simulink model "UnifiedPowerFlowController"  (R2024a)
settings: Solver=FixedStepDiscrete  StartTime=0.0  StopTime=0.8  FixedStep=Ts  RelTol=1e-3
PreLoadFcn:
  | Ts=1/512/60;
undefined symbols (not defined in the file or in its folder): DiscIntNeverNeededParam
libraries: spsabctodq0Lib x10, spsMeanVariableFrequencyLib x10, spsThreeLevelBridgeLib x8, spsVoltageMeasurementLib x8, spsZigzagPhaseShiftingTransformerLib x8, spsCurrentMeasurementLib x6, spsSecondOrderFilterLib x5, spsThreePhaseVIMeasurementLib x4, spsSeriesRLCBranchLib x4, spsDistributedParametersLineLib x3, spsPowerPositiveSequenceLib x3, spsThreePhaseSourceLib x2
(part 3 of 7)

== system UnifiedPowerFlowController/UPFC Controller/SE Control (SSSC)/PLL1 ==
  Vabc (pu) : Inport  PortDimensions=3
  Constant4 : Constant  Value=2*pi
  Correction for delay : Gain  Gain=Nstep*Ts*2*pi  SaturateOnIntegerOverflow=on  OutDataTypeStr=Inherit: Same as input  ParamDataTypeStr=Inherit: Same as input
  Discrete PI Controller : Subsystem  DialogController=POWERSYS.PowerSysDialog  mask(Discrete PI Controller){Kp=Kp, Ki=Ki, Par_Limits=2*pi*Finit*[1.25 0.75], Init=2*pi*Finit, Ts=Ts}
      mask prompts: Kp "Proportional gain (Kp):"; Ki "Integral gain (Ki):"; Par_Limits "Output limits: [ Upper   Lower ]"; Init "Output initial value:"; Ts "Sample time:"
      mask help: This block implements a discrete PI controller.
      mask init:
      | UpperLimit=Par_Limits(1);
      | LowerLimit=Par_Limits(2);
      | power_initmask();
      mask Help: This block is part of a subset of blocks in the Extras library that does not have documentation associated with it, other than the block mask description.
      mask Display: disp('PI');
  Discrete Rate Limiter : Subsystem  DialogController=POWERSYS.PowerSysDialog  mask(Discrete Rate Limiter){R=10, F=-10, Vinit=Finit, Ts=Ts}
      mask prompts: R "Rising slew rate:"; F "Falling slew rate:"; Vinit "Initial input:"; Ts "Sample time:"
      mask help: DISCRETE BLOCK : Limit rising and falling rates of signal
      mask init:
      | UpperLimit=R*Ts;
      | LowerLimit=F*Ts;
      | power_initmask();
      mask Help: This block is part of a subset of blocks in the Extras library that does not have documentation associated with it, other than the block mask description.
      mask Display: disp('Discrete\nRate\nLimiter')
  Discrete-Time Integrator : DiscreteIntegrator  InitialCondition=Phase_Init*pi/180  SampleTime=Ts  ICPrevOutput=DiscIntNeverNeededParam  ICPrevScaledInput=DiscIntNeverNeededParam
  Gain10 : Gain  Gain=1/2/pi  SaturateOnIntegerOverflow=on  OutDataTypeStr=Inherit: Same as input  ParamDataTypeStr=Inherit: Same as input
  Math Function : Math  Operator=mod  SignedPower=on
  Mean (Variable Frequency) : spsMeanVariableFrequencyLib/Mean (Variable Frequency)  Finit=Finit  Fmin=45  Vinit=0  Ts=Ts
  Second-Order Filter : spsSecondOrderFilterLib/Second-Order Filter  FilterType=Lowpass  Fo=25  Zeta=0.707  Ts=Ts  Initialize=on  Vac_Init=[0 -25 60]  Vdc_Init=Finit  PlotResponse=off  FreqRange=[0, 500, 1]
  Selector : Selector  InputPortWidth=3  IndexOptions=Index vector (dialog)  Indices=2  OutputSizes=1
  Sum : Sum  InputSameDT=on  SaturateOnIntegerOverflow=on  OutDataTypeStr=Inherit: Same as first input
  Unit Delay : UnitDelay  InitialCondition=Finit  SampleTime=Ts  HasFrameUpgradeWarning=on
  abc to dq0 : spsabctodq0Lib/abc to dq0  Alignment=90 degrees behind phase A axis
  Freq : Outport  VectorParamsAs1DForOutWhenUnconnected=off
  wt : Outport  Port=2  VectorParamsAs1DForOutWhenUnconnected=off
  wires:
  Sum/1 -> wt/1
  Selector/1 -> Mean (Variable Frequency)/2  "Vq"
  Second-Order Filter/1 -> Unit Delay/1
  Unit Delay/1 -> Correction for delay/1, Mean (Variable Frequency)/1, Freq/1
  Discrete Rate Limiter/1(Out) -> Second-Order Filter/1
  Gain10/1 -> Discrete Rate Limiter/1(In)
  Discrete PI Controller/1(Out) -> Gain10/1, Discrete-Time Integrator/1  "W"
  Math Function/1 -> abc to dq0/2, Sum/2
  Discrete-Time Integrator/1 -> Math Function/1
  Constant4/1 -> Math Function/2
  abc to dq0/1 -> Selector/1
  Vabc (pu)/1 -> abc to dq0/1
  Mean (Variable Frequency)/1 -> Discrete PI Controller/1(Error)
  Correction for delay/1 -> Sum/1

== system UnifiedPowerFlowController/UPFC Controller/SE Control (SSSC)/determine +pi//2 or -pi//2 phase shift ==
  Vref : Inport
  Delta_Alpha : Inport  Port=2
  Constant1 : Constant  Value=pi/2
  Product : Product  SaturateOnIntegerOverflow=on  OutDataTypeStr=Inherit: Same as first input
  Sum1 : Sum  SaturateOnIntegerOverflow=on
  Switch : Switch  InputSameDT=off
  Vdcmin1 : Constant
  Vdcmin2 : Constant  Value=-1
  Alpha : Outport  VectorParamsAs1DForOutWhenUnconnected=off
  wires:
  Product/1 -> Alpha/1
  Sum1/1 -> Product/2
  Switch/1 -> Product/1
  Vdcmin2/1 -> Switch/3
  Delta_Alpha/1 -> Sum1/2
  Vref/1 -> Switch/2
  Vdcmin1/1 -> Switch/1
  Constant1/1 -> Sum1/1

== system UnifiedPowerFlowController/UPFC Controller/SE Control (UPFC)/Current Regulators ==
  note: Current Regulators
  note: =================
  Id_Iq_Ref : Inport  PortDimensions=2
  Id_Iq : Inport  Port=2  PortDimensions=2
  Demux : Demux  Outputs=2
      settings: DisplayOption=none
  Demux1 : Demux  Outputs=2
      settings: DisplayOption=none
  Id PID : Subsystem  DialogController=POWERSYS.PowerSysDialog  mask(Discrete PID Controller){Kp=Kp, Ki=Ki, Kd=Kd, TcD=TcD, Par_Limits=Par_Limits, Init=Init, Ts=Ts}
      mask prompts: Kp "Proportional gain (Kp):"; Ki "Integral gain (Ki):"; Kd "Derivative gain (Kd):"; TcD "Time constant for derivative (s):"; Par_Limits "Output limits: [ Upper   Lower ]"; Init "Output initial value:"; Ts "Sample time:"
      mask help: This block implements a discrete PID controller.
      mask init:
      | UpperLimit=Par_Limits(1);
      | LowerLimit=Par_Limits(2);
      | power_initmask();
      mask Help: This block is part of a subset of blocks in the Extras library that does not have documentation associated with it, other than the block mask description.
      mask Display: disp('PID');
  Id PID1 : Subsystem  DialogController=POWERSYS.PowerSysDialog  mask(Discrete PID Controller){Kp=Kp, Ki=Ki, Kd=Kd, TcD=TcD, Par_Limits=Par_Limits, Init=Init, Ts=Ts}
      mask prompts: Kp "Proportional gain (Kp):"; Ki "Integral gain (Ki):"; Kd "Derivative gain (Kd):"; TcD "Time constant for derivative (s):"; Par_Limits "Output limits: [ Upper   Lower ]"; Init "Output initial value:"; Ts "Sample time:"
      mask help: This block implements a discrete PID controller.
      mask init:
      | UpperLimit=Par_Limits(1);
      | LowerLimit=Par_Limits(2);
      | power_initmask();
      mask Help: This block is part of a subset of blocks in the Extras library that does not have documentation associated with it, other than the block mask description.
      mask Display: disp('PID');
  Mux : Mux  Inputs=2
  Sum : Sum  Inputs=|-+  InputSameDT=on  SaturateOnIntegerOverflow=on  OutDataTypeStr=Inherit: Same as first input
  Sum1 : Sum  Inputs=|-+  InputSameDT=on  SaturateOnIntegerOverflow=on  OutDataTypeStr=Inherit: Same as first input
  VdVq* : Outport  VectorParamsAs1DForOutWhenUnconnected=off
  wires:
  Id_Iq/1 -> Demux/1
  Demux/1 -> Sum/1  "Id"
  Demux1/1 -> Sum/2  "Id_Ref"
  Demux/2 -> Sum1/1  "Iq"
  Sum1/1 -> Id PID1/1(Error)
  Demux1/2 -> Sum1/2  "Iq_Ref"
  Id_Iq_Ref/1 -> Demux1/1
  Mux/1 -> VdVq*/1
  Id PID/1(Out) -> Mux/1  "Vd"
  Id PID1/1(Out) -> Mux/2  "Vq"
  Sum/1 -> Id PID/1(Error)

== system UnifiedPowerFlowController/UPFC Controller/SE Control (UPFC)/Firing Pulses Generator ==
  Sigma : Inport  PortDimensions=1
  D_Alpha : Inport  Port=2  PortDimensions=1
  Alpha : Inport  Port=3  PortDimensions=1
  wt : Inport  Port=4  PortDimensions=1
  " Deg->Rad" : Gain  Gain=pi/180  SaturateOnIntegerOverflow=on  OutDataTypeStr=Inherit: Same as input  ParamDataTypeStr=Inherit: Same as input
  Bridge 1D : Subsystem
  "Bridge 1Y " : Subsystem
  Bridge 2D : Subsystem
  Bridge 2Y : Subsystem
  Constant : Constant  Value=[0 -30 -15 -45]*pi/180 + 7.5*pi/180
  Deg->Rad : Gain  Gain=pi/180  SaturateOnIntegerOverflow=on  OutDataTypeStr=Inherit: Same as input  ParamDataTypeStr=Inherit: Same as input
  "Deg->Rad " : Gain  Gain=pi/180  SaturateOnIntegerOverflow=on  OutDataTypeStr=Inherit: Same as input  ParamDataTypeStr=Inherit: Same as input
  Demux : Demux
      settings: DisplayOption=none
  Mux : Mux  Inputs=[12 12 12 12]
  Sum : Sum  InputSameDT=on  SaturateOnIntegerOverflow=on  OutDataTypeStr=Inherit: Same as first input
  Pulses : Outport  VectorParamsAs1DForOutWhenUnconnected=off
  wires:
  Alpha/1 -> Deg->Rad/1
  Constant/1 -> Sum/2
  Sum/1 -> Demux/1
  "Bridge 1Y "/1(Pulses) -> Mux/1
  Mux/1 -> Pulses/1
  Demux/1 -> "Bridge 1Y "/1(wt)
  Sigma/1 -> "Deg->Rad "/1
  Demux/2 -> Bridge 1D/1(wt)
  Demux/3 -> Bridge 2Y/1(wt)
  Demux/4 -> Bridge 2D/1(wt)
  Deg->Rad/1 -> "Bridge 1Y "/2(Alpha), Bridge 1D/2(Alpha), Bridge 2Y/2(Alpha), Bridge 2D/2(Alpha)
  "Deg->Rad "/1 -> "Bridge 1Y "/3(Sigma), Bridge 1D/3(Sigma), Bridge 2Y/3(Sigma), Bridge 2D/3(Sigma)
  " Deg->Rad"/1 -> Bridge 2D/4(D_Alpha), Bridge 2Y/4(D_Alpha), Bridge 1D/4(D_Alpha), "Bridge 1Y "/4(D_Alpha)
  D_Alpha/1 -> " Deg->Rad"/1
  Bridge 1D/1(Pulses) -> Mux/2
  Bridge 2Y/1(Pulses) -> Mux/3
  Bridge 2D/1(Pulses) -> Mux/4
  wt/1 -> Sum/1

== system UnifiedPowerFlowController/UPFC Controller/SE Control (UPFC)/Mag//rho and sigma computation ==
  VdVq : Inport
  VdcPM_SE : Inport  Port=2  PortDimensions=2
  Demux : Demux  Outputs=2
      settings: DisplayOption=none
  Sigma Computation : Subsystem
  Sum1 : Sum  Inputs=1  InputSameDT=on  SaturateOnIntegerOverflow=on  OutDataTypeStr=Inherit: Same as first input
  Vd_Vq--> Mag,rho : Subsystem
  Sigma : Outport  VectorParamsAs1DForOutWhenUnconnected=off
  rho : Outport  Port=2  VectorParamsAs1DForOutWhenUnconnected=off
  tag scope: Mag_rho_SE=global, Sigma_SE=global
  wires:
  Demux/1 -> Sigma Computation/1(Mag (pu))
  VdcPM_SE/1 -> Sum1/1
  Vd_Vq--> Mag,rho/1(Mag_rho) -> Demux/1, [Mag_rho_SE]
  Sum1/1 -> Sigma Computation/2(Vdc (V))
  VdVq/1 -> Vd_Vq--> Mag,rho/1(Vd_Vq)
  Demux/2 -> rho/1
  Sigma Computation/1(sigma (deg)) -> Sigma/1, [Sigma_SE]

== system UnifiedPowerFlowController/UPFC Controller/SE Control (UPFC)/Measurement System ==
  Freq : Inport  PortDimensions=1
  wt : Inport  Port=2  PortDimensions=1
  Vabc : Inport  Port=3  PortDimensions=3
  Iabc : Inport  Port=4  PortDimensions=3
  PQ Computaion : Subsystem
  Selector : Selector  InputPortWidth=3  IndexOptions=Index vector (dialog)  Indices=[1 2]  OutputSizes=1
  Voltage Measurement : Subsystem  mask(Discrete 3-phase PLL-Driven Positive-Sequence Fundamental Value){Finit=60, Par_Init=[1.0001 -1.5], Ts=Ts}
      mask prompts: Finit "Initial fundamental frequency (Hz):"; Par_Init "Initial input (positive component): [ Mag  Phase-relative-to-PLL(degrees) ]"; Ts "Sample time:"
      mask help:
      | For a supplied fundamental frequency (port Freq), this discrete block computes  the positive-sequence component (Magnitude and Phase)  of a set of three balanced or unbalanced signals (port abc) which may contain harmonics.
      |  Input port "Sin_Cos" (a two-dimension signal) provides the reference frame required for the computation..
      |  First and second outputs return respectively the magnitude and phase (in degrees relative to the PLL phase)) of the fundamental.
      | For the first cycle of simulation, the outputs are held constant to the values specified by the parameter "Initial input".
      mask init:
      | Real_Init=Par_Init(1)*cos(pi/180*Par_Init(2));
      | Imag_Init=Par_Init(1)*sin(pi/180*Par_Init(2));
  Voltage Measurement1 : Subsystem  mask(Discrete 3-phase PLL-Driven Positive-Sequence Fundamental Value){Finit=60, Par_Init=[8.7 0], Ts=Ts}
      mask prompts: Finit "Initial fundamental frequency (Hz):"; Par_Init "Initial input (positive component): [ Mag  Phase-relative-to-PLL(degrees) ]"; Ts "Sample time:"
      mask help:
      | For a supplied fundamental frequency (port Freq), this discrete block computes  the positive-sequence component (Magnitude and Phase)  of a set of three balanced or unbalanced signals (port abc) which may contain harmonics.
      |  Input port "Sin_Cos" (a two-dimension signal) provides the reference frame required for the computation..
      |  First and second outputs return respectively the magnitude and phase (in degrees relative to the PLL phase)) of the fundamental.
      | For the first cycle of simulation, the outputs are held constant to the values specified by the parameter "Initial input".
      mask init:
      | Real_Init=Par_Init(1)*cos(pi/180*Par_Init(2));
      | Imag_Init=Par_Init(1)*sin(pi/180*Par_Init(2));
  abc to dq0 : spsabctodq0Lib/abc to dq0  Alignment=90 degrees behind phase A axis
  PQ : Outport  VectorParamsAs1DForOutWhenUnconnected=off
  Vd_Vq : Outport  Port=2  VectorParamsAs1DForOutWhenUnconnected=off
  Id_Iq : Outport  Port=3  VectorParamsAs1DForOutWhenUnconnected=off
  wires:
  Voltage Measurement/1(VdVq) -> Vd_Vq/1, PQ Computaion/1(Vd_Vq)
  Freq/1 -> Voltage Measurement/1(Freq), Voltage Measurement1/1(Freq)
  Iabc/1 -> Voltage Measurement1/3(abc), abc to dq0/1
  Vabc/1 -> Voltage Measurement/3(abc)
  PQ Computaion/1(P_Q) -> PQ/1
  abc to dq0/1 -> Selector/1
  Selector/1 -> Id_Iq/1
  Voltage Measurement1/1(IdIq) -> PQ Computaion/2(Id_Iq)
  wt/1 -> abc to dq0/2, Voltage Measurement1/2(wt), Voltage Measurement/2(wt)

== system UnifiedPowerFlowController/UPFC Controller/SE Control (UPFC)/PLL1 ==
  Vabc (pu) : Inport  PortDimensions=3
  Constant4 : Constant  Value=2*pi
  Correction for delay : Gain  Gain=Nstep*Ts*2*pi  SaturateOnIntegerOverflow=on  OutDataTypeStr=Inherit: Same as input  ParamDataTypeStr=Inherit: Same as input
  Discrete PI Controller : Subsystem  DialogController=POWERSYS.PowerSysDialog  mask(Discrete PI Controller){Kp=Kp, Ki=Ki, Par_Limits=2*pi*Finit*[1.25 0.75], Init=2*pi*Finit, Ts=Ts}
      mask prompts: Kp "Proportional gain (Kp):"; Ki "Integral gain (Ki):"; Par_Limits "Output limits: [ Upper   Lower ]"; Init "Output initial value:"; Ts "Sample time:"
      mask help: This block implements a discrete PI controller.
      mask init:
      | UpperLimit=Par_Limits(1);
      | LowerLimit=Par_Limits(2);
      | power_initmask();
      mask Help: This block is part of a subset of blocks in the Extras library that does not have documentation associated with it, other than the block mask description.
      mask Display: disp('PI');
  Discrete Rate Limiter : Subsystem  DialogController=POWERSYS.PowerSysDialog  mask(Discrete Rate Limiter){R=10, F=-10, Vinit=Finit, Ts=Ts}
      mask prompts: R "Rising slew rate:"; F "Falling slew rate:"; Vinit "Initial input:"; Ts "Sample time:"
      mask help: DISCRETE BLOCK : Limit rising and falling rates of signal
      mask init:
      | UpperLimit=R*Ts;
      | LowerLimit=F*Ts;
      | power_initmask();
      mask Help: This block is part of a subset of blocks in the Extras library that does not have documentation associated with it, other than the block mask description.
      mask Display: disp('Discrete\nRate\nLimiter')
  Discrete-Time Integrator : DiscreteIntegrator  InitialCondition=Phase_Init*pi/180  SampleTime=Ts  ICPrevOutput=DiscIntNeverNeededParam  ICPrevScaledInput=DiscIntNeverNeededParam
  Gain10 : Gain  Gain=1/2/pi  SaturateOnIntegerOverflow=on  OutDataTypeStr=Inherit: Same as input  ParamDataTypeStr=Inherit: Same as input
  Math Function : Math  Operator=mod  SignedPower=on
  Mean (Variable Frequency) : spsMeanVariableFrequencyLib/Mean (Variable Frequency)  Finit=Finit  Fmin=45  Vinit=0  Ts=Ts
  Second-Order Filter : spsSecondOrderFilterLib/Second-Order Filter  FilterType=Lowpass  Fo=25  Zeta=0.707  Ts=Ts  Initialize=on  Vac_Init=[0 -25 60]  Vdc_Init=Finit  PlotResponse=off  FreqRange=[0, 500, 1]
  Selector : Selector  InputPortWidth=3  IndexOptions=Index vector (dialog)  Indices=2  OutputSizes=1
  Sum : Sum  InputSameDT=on  SaturateOnIntegerOverflow=on  OutDataTypeStr=Inherit: Same as first input
  Unit Delay : UnitDelay  InitialCondition=Finit  SampleTime=Ts  HasFrameUpgradeWarning=on
  abc to dq0 : spsabctodq0Lib/abc to dq0  Alignment=90 degrees behind phase A axis
  Freq : Outport  VectorParamsAs1DForOutWhenUnconnected=off
  wt : Outport  Port=2  VectorParamsAs1DForOutWhenUnconnected=off
  wires:
  Sum/1 -> wt/1
  Selector/1 -> Mean (Variable Frequency)/2  "Vq"
  Second-Order Filter/1 -> Unit Delay/1
  Unit Delay/1 -> Correction for delay/1, Mean (Variable Frequency)/1, Freq/1
  Discrete Rate Limiter/1(Out) -> Second-Order Filter/1
  Gain10/1 -> Discrete Rate Limiter/1(In)
  Discrete PI Controller/1(Out) -> Gain10/1, Discrete-Time Integrator/1  "W"
  Math Function/1 -> abc to dq0/2, Sum/2
  Discrete-Time Integrator/1 -> Math Function/1
  Constant4/1 -> Math Function/2
  abc to dq0/1 -> Selector/1
  Vabc (pu)/1 -> abc to dq0/1
  Mean (Variable Frequency)/1 -> Discrete PI Controller/1(Error)
  Correction for delay/1 -> Sum/1

== system UnifiedPowerFlowController/UPFC Controller/SE Control (UPFC)/Reference Computation ==
  note: Iq* = ( P*Vq - Q*Vd ) / ( Vd^2 + Vq^2 )
  note: Id* = ( P*Vd + Q*Vq ) / ( Vd^2 + Vq^2 )
  note: Reference computation:
  note: 0.25pu/cycle
  note: 0.25pu/cycle
  Pref_Qref : Inport  PortDimensions=2
  Vd_Vq : Inport  Port=2  PortDimensions=2
  Constant : Constant  Value=1e-6
  Constant1 : Constant  Value=0
  Demux1 : Demux  Outputs=2
      settings: DisplayOption=none
  Demux2 : Demux  Outputs=2
      settings: DisplayOption=none
  Fcn3 : Fcn  Expr=u[1]*u[1]+u[2]*u[2]
  Mux3 : Mux  Inputs=2
  Product{2..5} (4 alike) : Product  InputSameDT=on  SaturateOnIntegerOverflow=on  OutDataTypeStr=Inherit: Same as first input
  Product6 : Product  Inputs=*/  InputSameDT=on  SaturateOnIntegerOverflow=on  OutDataTypeStr=Inherit: Same as first input
  "Rate Limiter " : Subsystem  DialogController=POWERSYS.PowerSysDialog  mask(Discrete Rate Limiter){R=10, F=-10, Vinit=8.7, Ts=Ts}
      mask prompts: R "Rising slew rate:"; F "Falling slew rate:"; Vinit "Initial input:"; Ts "Sample time:"
      mask help: DISCRETE BLOCK : Limit rising and falling rates of signal
      mask init:
      | UpperLimit=R*Ts;
      | LowerLimit=F*Ts;
      | power_initmask();
      mask Help: This block is part of a subset of blocks in the Extras library that does not have documentation associated with it, other than the block mask description.
      mask Display: disp('Discrete\nRate\nLimiter')
  "Rate Limiter  " : Subsystem  DialogController=POWERSYS.PowerSysDialog  mask(Discrete Rate Limiter){R=0.25*60, F=-0.25*60, Vinit=-0.6, Ts=Ts}
      mask prompts: R "Rising slew rate:"; F "Falling slew rate:"; Vinit "Initial input:"; Ts "Sample time:"
      mask help: DISCRETE BLOCK : Limit rising and falling rates of signal
      mask init:
      | UpperLimit=R*Ts;
      | LowerLimit=F*Ts;
      | power_initmask();
      mask Help: This block is part of a subset of blocks in the Extras library that does not have documentation associated with it, other than the block mask description.
      mask Display: disp('Discrete\nRate\nLimiter')
  Relational Operator : RelationalOperator  Operator=~=
  Sum : Sum  InputSameDT=on  SaturateOnIntegerOverflow=on  OutDataTypeStr=Inherit: Same as first input
  Sum1 : Sum  Inputs=+-  InputSameDT=on  SaturateOnIntegerOverflow=on  OutDataTypeStr=Inherit: Same as first input
  Switch : Switch  Threshold=0.5
  Id*_Iq* : Outport  VectorParamsAs1DForOutWhenUnconnected=off
  wires:
  Pref_Qref/1 -> Demux2/1
  Demux1/1 -> Product5/2, Product2/1
  Demux1/2 -> Product4/2, Product3/1
  Product4/1 -> Sum1/1
  Product2/1 -> Sum/1
  Product3/1 -> Sum/2
  Sum1/1 -> Mux3/2
  Product5/1 -> Sum1/2
  Switch/1 -> Product6/2
  Relational Operator/1 -> Switch/2
  Fcn3/1 -> Relational Operator/1, Switch/1
  Constant1/1 -> Relational Operator/2
  Constant/1 -> Switch/3
  Vd_Vq/1 -> Fcn3/1, Demux1/1
  Product6/1 -> Id*_Iq*/1
  Mux3/1 -> Product6/1
  Sum/1 -> Mux3/1
  Demux2/1 -> "Rate Limiter "/1(In)
  "Rate Limiter "/1(Out) -> Product4/1, Product2/2
  Demux2/2 -> "Rate Limiter  "/1(In)
  "Rate Limiter  "/1(Out) -> Product5/1, Product3/2

== system UnifiedPowerFlowController/UPFC Controller/SE Control (UPFC)/Vd,Vq Selection (Auto//Man) and Limit Computation ==
  VdVq* : Inport  PortDimensions=2
  OpMode : Inport  Port=2  PortDimensions=1
  Constant10 : Constant  Value=rhoInj
  Constant9 : Constant  Value=MagInj
  Mag_ramp (pu) : Constant  Value=0.1
  Switch2 : Switch  Threshold=0.5
  Switch3 : Switch  Threshold=0.5
  Vd,Vq Selection and Limit Computation : Subsystem
  rho_ramp (deg) : simulink/Sources/Ramp  slope=90  start=0.5  InitialOutput=0
  VdVq_inj : Outport  VectorParamsAs1DForOutWhenUnconnected=off
  wires:
  OpMode/1 -> Vd,Vq Selection and Limit Computation/2(OpMode)
  Switch2/1 -> Vd,Vq Selection and Limit Computation/4(rho* (man))
  Switch3/1 -> Vd,Vq Selection and Limit Computation/3(Mag* (man))
  Constant9/1 -> Switch3/3
  Constant10/1 -> Switch2/3
  rho_ramp (deg)/1 -> Switch2/1
  Mag_ramp (pu)/1 -> Switch3/1
  VdVq*/1 -> Vd,Vq Selection and Limit Computation/1(Vd_Vq(auto)*)
  Vd,Vq Selection and Limit Computation/1(VdVq) -> VdVq_inj/1
  [rhoRamp_On] -> Switch3/2, Switch2/2

== system UnifiedPowerFlowController/UPFC Controller/SH Control (STATCOM)/Current Regulator ==
  Iq_Ref : Inport
  Iq : Inport  Port=2
  Discrete PI Controller : Subsystem  DialogController=POWERSYS.PowerSysDialog  mask(Discrete PI Controller){Kp=Kp, Ki=Ki, Par_Limits=[ UpperLimit  LowerLimit ]*10, Init=Init, Ts=Ts}
      mask prompts: Kp "Proportional gain (Kp):"; Ki "Integral gain (Ki):"; Par_Limits "Output limits: [ Upper   Lower ]"; Init "Output initial value:"; Ts "Sample time:"
      mask help: This block implements a discrete PI controller.
      mask init:
      | UpperLimit=Par_Limits(1);
      | LowerLimit=Par_Limits(2);
      | power_initmask();
      mask Help: This block is part of a subset of blocks in the Extras library that does not have documentation associated with it, other than the block mask description.
      mask Display: disp('PI');
  Sum : Sum  Inputs=-+|  InputSameDT=on  SaturateOnIntegerOverflow=on  OutDataTypeStr=Inherit: Same as first input
  Alpha : Outport  InitialOutput=0  VectorParamsAs1DForOutWhenUnconnected=off
  wires:
  Sum/1 -> Discrete PI Controller/1(Error)  "Err"
  Iq/1 -> Sum/2
  Iq_Ref/1 -> Sum/1
  Discrete PI Controller/1(Out) -> Alpha/1

== system UnifiedPowerFlowController/UPFC Controller/SH Control (STATCOM)/DC Balance Regulator ==
  Iq_avg : Inport  PortDimensions=1
  +/-Vdc/2 : Inport  Port=2  PortDimensions=2
  Abs : Abs
  D_Alpha(Manual) : Constant  Value=0
  D_Alpha1 : Constant  Value=0
  D_Alpha2 : Constant  Value=0
  D_Alpha5 : Constant  Value=0.1
  Demux : Demux  Outputs=2
      settings: DisplayOption=none
  Gain : Gain  Gain=0  SaturateOnIntegerOverflow=on  OutDataTypeStr=Inherit: Same as input  ParamDataTypeStr=Inherit: Same as input
  Gain1 : Gain  Gain=-1  SaturateOnIntegerOverflow=on  OutDataTypeStr=Inherit: Same as input  ParamDataTypeStr=Inherit: Same as input
  Mean : spsMeanLib/Mean  Freq=60  Vinit=0  Ts=Ts
  Mode : Constant
  Multiport Switch : MultiPortSwitch
  PI Regulator : Subsystem  mask(Discrete PI Controller){Kp=0.001, Ki=0.01, Par_Limits=[2 -2], Init=0, Ts=Ts}
      mask prompts: Kp "Proportional gain (Kp):"; Ki "Integral gain (Ki):"; Par_Limits "Output limits: [ Upper   Lower ]"; Init "Output initial value:"; Ts "Sample time:"
      mask help: This block implements a discrete PI controller.
      mask init:
      | UpperLimit=Par_Limits(1);
      | LowerLimit=Par_Limits(2);
      mask Display: disp('PI');
  Relational Operator : RelationalOperator  Operator=<=
  Relational Operator1 : RelationalOperator  Operator=<
  Sum2 : Sum  Inputs=-+  InputSameDT=on  SaturateOnIntegerOverflow=on  OutDataTypeStr=Inherit: Same as first input
  Switch : Switch  Threshold=0.5
  Switch1 : Switch  Threshold=0.5
  D_Alpha : Outport  VectorParamsAs1DForOutWhenUnconnected=off
  wires:
  Demux/2 -> Sum2/2
  Demux/1 -> Sum2/1
  +/-Vdc/2/1 -> Demux/1
  Iq_avg/1 -> Relational Operator/1, Abs/1
  Sum2/1 -> Mean/1
  Switch1/1 -> PI Regulator/1(Error)
  Gain/1 -> Switch1/1
  Mean/1 -> Gain/1, Switch1/3
  D_Alpha1/1 -> Relational Operator/2
  Abs/1 -> Relational Operator1/1
  D_Alpha5/1 -> Relational Operator1/2
  Gain1/1 -> Switch/3
  Relational Operator/1 -> Switch/2
  Switch/1 -> Multiport Switch/2  "Auto"
  D_Alpha2/1 -> Multiport Switch/4  "Off"
  Mode/1 -> Multiport Switch/1
  PI Regulator/1(Out) -> Switch/1, Gain1/1
  D_Alpha(Manual)/1 -> Multiport Switch/3  "Man"
  Multiport Switch/1 -> D_Alpha/1
  Relational Operator1/1 -> Switch1/2, PI Regulator/2(Reset)

== system UnifiedPowerFlowController/UPFC Controller/SH Control (STATCOM)/Firing Pulses Generator ==
  Alpha : Inport  PortDimensions=1
  Sigma : Inport  Port=2  PortDimensions=1
  wt : Inport  Port=3  PortDimensions=1
  D_Alpha : Inport  Port=4  PortDimensions=1
  " Deg->Rad" : Gain  Gain=pi/180  SaturateOnIntegerOverflow=on  OutDataTypeStr=Inherit: Same as input  ParamDataTypeStr=Inherit: Same as input
  Bridge 1D : Subsystem
  "Bridge 1Y " : Subsystem
  Bridge 2D : Subsystem
  Bridge 2Y : Subsystem
  Constant : Constant  Value=[0 -30 -15 -45]*pi/180 + 7.5*pi/180
  Deg->Rad : Gain  Gain=pi/180  SaturateOnIntegerOverflow=on  OutDataTypeStr=Inherit: Same as input  ParamDataTypeStr=Inherit: Same as input
  "Deg->Rad " : Gain  Gain=pi/180  SaturateOnIntegerOverflow=on  OutDataTypeStr=Inherit: Same as input  ParamDataTypeStr=Inherit: Same as input
  Demux : Demux
      settings: DisplayOption=none
  Mux : Mux  Inputs=[12 12 12 12]
  Sum : Sum  InputSameDT=on  SaturateOnIntegerOverflow=on  OutDataTypeStr=Inherit: Same as first input
  Pulses : Outport  VectorParamsAs1DForOutWhenUnconnected=off
  wires:
  Alpha/1 -> Deg->Rad/1
  Constant/1 -> Sum/2
  Sum/1 -> Demux/1
  "Bridge 1Y "/1(Pulses) -> Mux/1
  Mux/1 -> Pulses/1
  Demux/1 -> "Bridge 1Y "/1(wt)
  Sigma/1 -> "Deg->Rad "/1
  Demux/2 -> Bridge 1D/1(wt)
  Demux/3 -> Bridge 2Y/1(wt)
  Demux/4 -> Bridge 2D/1(wt)
  Deg->Rad/1 -> "Bridge 1Y "/2(Alpha), Bridge 1D/2(Alpha), Bridge 2Y/2(Alpha), Bridge 2D/2(Alpha)
  "Deg->Rad "/1 -> "Bridge 1Y "/3(Sigma), Bridge 1D/3(Sigma), Bridge 2Y/3(Sigma), Bridge 2D/3(Sigma)
  " Deg->Rad"/1 -> Bridge 2D/4(D_Alpha), Bridge 2Y/4(D_Alpha), Bridge 1D/4(D_Alpha), "Bridge 1Y "/4(D_Alpha)
  D_Alpha/1 -> " Deg->Rad"/1
  Bridge 1D/1(Pulses) -> Mux/2
  Bridge 2Y/1(Pulses) -> Mux/3
  Bridge 2D/1(Pulses) -> Mux/4
  wt/1 -> Sum/1

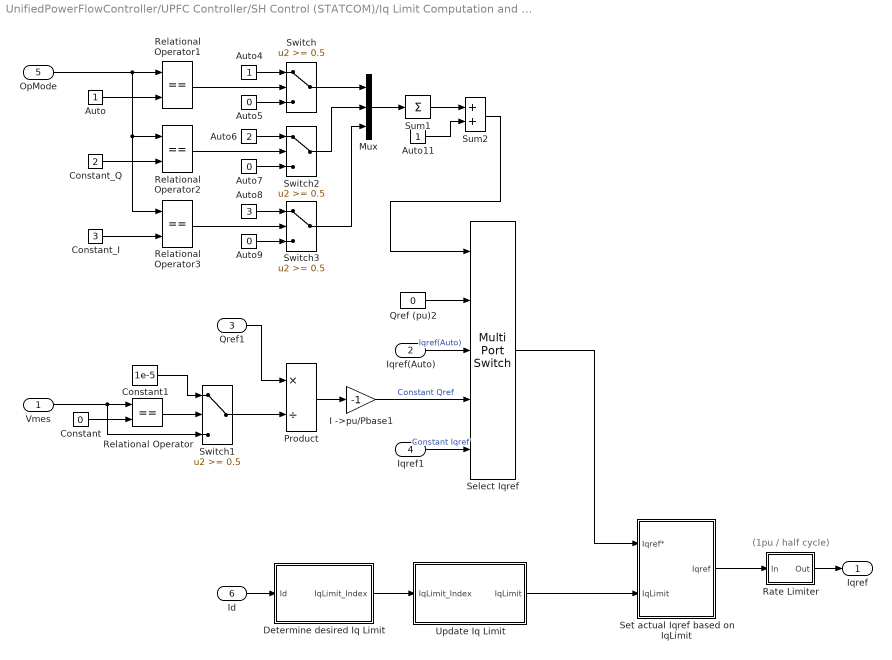
== system UnifiedPowerFlowController/UPFC Controller/SH Control (STATCOM)/Iq Limit Computation and Iqref Selection ==
  note: (1pu / half cycle)
  Vmes : Inport
  Iqref(Auto) : Inport  Port=2
  Qref1 : Inport  Port=3
  Iqref1 : Inport  Port=4
  OpMode : Inport  Port=5
  Id : Inport  Port=6
  Auto : Constant
  Auto11 : Constant
  Auto4 : Constant
  Auto5 : Constant  Value=0
  Auto6 : Constant  Value=2
  Auto7 : Constant  Value=0
  Auto8 : Constant  Value=3
  Auto9 : Constant  Value=0
  Constant : Constant  Value=0
  Constant1 : Constant  Value=1e-5
  Constant_I : Constant  Value=3
  Constant_Q : Constant  Value=2
  Determine desired Iq Limit : Subsystem
  I ->pu/Pbase1 : Gain  Gain=-1  SaturateOnIntegerOverflow=on  OutDataTypeStr=Inherit: Same as input  ParamDataTypeStr=Inherit: Same as input
  Mux : Mux  Inputs=3
  Product : Product  Inputs=*/  InputSameDT=on  SaturateOnIntegerOverflow=on  OutDataTypeStr=Inherit: Same as first input
  Qref (pu)2 : Constant  Value=0
  "Rate Limiter " : Subsystem  DialogController=POWERSYS.PowerSysDialog  mask(Discrete Rate Limiter){R=120, F=-120, Vinit=-0.33, Ts=Ts}
      mask prompts: R "Rising slew rate:"; F "Falling slew rate:"; Vinit "Initial input:"; Ts "Sample time:"
      mask help: DISCRETE BLOCK : Limit rising and falling rates of signal
      mask init:
      | UpperLimit=R*Ts;
      | LowerLimit=F*Ts;
      | power_initmask();
      mask Help: This block is part of a subset of blocks in the Extras library that does not have documentation associated with it, other than the block mask description.
      mask Display: disp('Discrete\nRate\nLimiter')
  Relational Operator{,1..3} (4 alike) : RelationalOperator  Operator===
  Select Iqref : MultiPortSwitch  Inputs=4
  Set actual Iqref based on IqLimit : Subsystem
  Sum1 : Sum  Inputs=1  InputSameDT=on  SaturateOnIntegerOverflow=on  OutDataTypeStr=Inherit: Same as first input
  Sum2 : Sum  InputSameDT=on  SaturateOnIntegerOverflow=on  OutDataTypeStr=Inherit: Same as first input
  Switch{,1..3} (4 alike) : Switch  Threshold=0.5
  Update Iq Limit : Subsystem
  Iqref : Outport  VectorParamsAs1DForOutWhenUnconnected=off
  wires:
  Switch2/1 -> Mux/2
  Auto11/1 -> Sum2/2
  Sum1/1 -> Sum2/1
  Switch3/1 -> Mux/3
  Mux/1 -> Sum1/1
  Switch/1 -> Mux/1
  Auto9/1 -> Switch3/3
  Auto8/1 -> Switch3/1
  Relational Operator3/1 -> Switch3/2
  Auto7/1 -> Switch2/3
  Auto6/1 -> Switch2/1
  Relational Operator2/1 -> Switch2/2
  Auto5/1 -> Switch/3
  Auto4/1 -> Switch/1
  Relational Operator1/1 -> Switch/2
  OpMode/1 -> Relational Operator3/1, Relational Operator2/1, Relational Operator1/1
  Constant_I/1 -> Relational Operator3/2
  Constant_Q/1 -> Relational Operator2/2
  Auto/1 -> Relational Operator1/2
  Sum2/1 -> Select Iqref/1
  Vmes/1 -> Relational Operator/1, Switch1/3
  Qref1/1 -> Product/1
  Relational Operator/1 -> Switch1/2
  Constant1/1 -> Switch1/1
  Switch1/1 -> Product/2
  Constant/1 -> Relational Operator/2
  Product/1 -> I ->pu/Pbase1/1
  Iqref1/1 -> Select Iqref/5  "Constant Iqref"
  Iqref(Auto)/1 -> Select Iqref/3  "Iqref(Auto)"
  I ->pu/Pbase1/1 -> Select Iqref/4  "Constant Qref"
  Qref (pu)2/1 -> Select Iqref/2
  Select Iqref/1 -> Set actual Iqref based on IqLimit/1(Iqref*)
  Determine desired Iq Limit/1(IqLimit_Index) -> Update Iq Limit/1(IqLimit_Index)
  Update Iq Limit/1(IqLimit) -> Set actual Iqref based on IqLimit/2(IqLimit)
  Set actual Iqref based on IqLimit/1(Iqref) -> "Rate Limiter "/1(In)
  "Rate Limiter "/1(Out) -> Iqref/1
  Id/1 -> Determine desired Iq Limit/1(Id)

== system UnifiedPowerFlowController/UPFC Controller/SH Control (STATCOM)/Measurement System ==
  Vabc : Inport  PortDimensions=3
  Iabc : Inport  Port=2  PortDimensions=3
  Freq : Inport  Port=3  PortDimensions=1
  wt : Inport  Port=4  PortDimensions=1
  Mean (Variable Frequency) : spsMeanVariableFrequencyLib/Mean (Variable Frequency)  Finit=60  Fmin=45  Vinit=0  Ts=Ts
  PQ Computaion : Subsystem
  Second-Order Filter : spsSecondOrderFilterLib/Second-Order Filter  FilterType=Lowpass  Fo=1200  Zeta=0.707  Ts=Ts  Initialize=off  Vac_Init="[0,  0,  60]"  Vdc_Init=0  PlotResponse=off  FreqRange=[0, 500, 1]
  Second-Order Filter1 : spsSecondOrderFilterLib/Second-Order Filter  FilterType=Lowpass  Fo=1200  Zeta=0.707  Ts=Ts  Initialize=off  Vac_Init="[0,  0,  60]"  Vdc_Init=0  PlotResponse=off  FreqRange=[0, 500, 1]
  Selector : Selector  InputPortWidth=2  IndexOptions=Index vector (dialog)  Indices=2  OutputSizes=1
  Selector1 : Selector  InputPortWidth=2  IndexOptions=Index vector (dialog)  Indices=1  OutputSizes=1
  Selector2 : Selector  InputPortWidth=3  IndexOptions=Index vector (dialog)  Indices=1:2  OutputSizes=1
  Voltage measurement (Positive sequence) : Subsystem  mask(Discrete 3-phase PLL-Driven Positive-Sequence Fundamental Value){Finit=60, Par_Init=[1 0], Ts=Ts}
      mask prompts: Finit "Initial fundamental frequency (Hz):"; Par_Init "Initial input (positive component): [ Mag  Phase-relative-to-PLL(degrees) ]"; Ts "Sample time:"
      mask help:
      | For a supplied fundamental frequency (port Freq), this discrete block computes  the positive-sequence component (Magnitude and Phase)  of a set of three balanced or unbalanced signals (port abc) which may contain harmonics.
      |  Input port "Sin_Cos" (a two-dimension signal) provides the reference frame required for the computation..
      |  First and second outputs return respectively the magnitude and phase (in degrees relative to the PLL phase)) of the fundamental.
      | For the first cycle of simulation, the outputs are held constant to the values specified by the parameter "Initial input".
      mask init:
      | Real_Init=Par_Init(1)*cos(pi/180*Par_Init(2));
      | Imag_Init=Par_Init(1)*sin(pi/180*Par_Init(2));
  abc to dq0 : spsabctodq0Lib/abc to dq0  Alignment=90 degrees behind phase A axis
  Vmes : Outport  VectorParamsAs1DForOutWhenUnconnected=off
  PQ : Outport  Port=2  VectorParamsAs1DForOutWhenUnconnected=off
  Iq : Outport  Port=3  VectorParamsAs1DForOutWhenUnconnected=off
  Iq_avg : Outport  Port=4  VectorParamsAs1DForOutWhenUnconnected=off
  Id : Outport  Port=5  VectorParamsAs1DForOutWhenUnconnected=off
  wires:
  Second-Order Filter/1 -> Id/1
  Selector1/1 -> Second-Order Filter/1
  Mean (Variable Frequency)/1 -> Iq_avg/1
  Selector/1 -> Second-Order Filter1/1, Mean (Variable Frequency)/2
  Freq/1 -> Mean (Variable Frequency)/1, PQ Computaion/3(Freq), Voltage measurement (Positive sequence)/2(Freq)
  abc to dq0/1 -> Selector2/1
  PQ Computaion/1(PQ(pu)) -> PQ/1
  wt/1 -> Voltage measurement (Positive sequence)/3(wt), abc to dq0/2
  Vabc/1 -> Voltage measurement (Positive sequence)/1(abc)
  Voltage measurement (Positive sequence)/1(Mag) -> Vmes/1  "Vmes"
  Voltage measurement (Positive sequence)/2(VdVq) -> PQ Computaion/1(Vd_Vq)
  Second-Order Filter1/1 -> Iq/1
  Iabc/1 -> abc to dq0/1
  Selector2/1 -> Selector1/1, Selector/1, PQ Computaion/2(Id_Iq)

== system UnifiedPowerFlowController/UPFC Controller/SH Control (STATCOM)/PLL ==
  Vabc (pu) : Inport  PortDimensions=3
  Constant4 : Constant  Value=2*pi
  Correction for delay : Gain  Gain=Nstep*Ts*2*pi  SaturateOnIntegerOverflow=on  OutDataTypeStr=Inherit: Same as input  ParamDataTypeStr=Inherit: Same as input
  Discrete PI Controller : Subsystem  DialogController=POWERSYS.PowerSysDialog  mask(Discrete PI Controller){Kp=Kp, Ki=Ki, Par_Limits=2*pi*Finit*[1.25 0.75], Init=2*pi*Finit, Ts=Ts}
      mask prompts: Kp "Proportional gain (Kp):"; Ki "Integral gain (Ki):"; Par_Limits "Output limits: [ Upper   Lower ]"; Init "Output initial value:"; Ts "Sample time:"
      mask help: This block implements a discrete PI controller.
      mask init:
      | UpperLimit=Par_Limits(1);
      | LowerLimit=Par_Limits(2);
      | power_initmask();
      mask Help: This block is part of a subset of blocks in the Extras library that does not have documentation associated with it, other than the block mask description.
      mask Display: disp('PI');
  Discrete Rate Limiter : Subsystem  DialogController=POWERSYS.PowerSysDialog  mask(Discrete Rate Limiter){R=10, F=-10, Vinit=Finit, Ts=Ts}
      mask prompts: R "Rising slew rate:"; F "Falling slew rate:"; Vinit "Initial input:"; Ts "Sample time:"
      mask help: DISCRETE BLOCK : Limit rising and falling rates of signal
      mask init:
      | UpperLimit=R*Ts;
      | LowerLimit=F*Ts;
      | power_initmask();
      mask Help: This block is part of a subset of blocks in the Extras library that does not have documentation associated with it, other than the block mask description.
      mask Display: disp('Discrete\nRate\nLimiter')
  Discrete-Time Integrator : DiscreteIntegrator  InitialCondition=Phase_Init*pi/180  SampleTime=Ts  ICPrevOutput=DiscIntNeverNeededParam  ICPrevScaledInput=DiscIntNeverNeededParam
  Gain10 : Gain  Gain=1/2/pi  SaturateOnIntegerOverflow=on  OutDataTypeStr=Inherit: Same as input  ParamDataTypeStr=Inherit: Same as input
  Math Function : Math  Operator=mod  SignedPower=on
  Mean (Variable Frequency) : spsMeanVariableFrequencyLib/Mean (Variable Frequency)  Finit=Finit  Fmin=45  Vinit=0  Ts=Ts
  Second-Order Filter : spsSecondOrderFilterLib/Second-Order Filter  FilterType=Lowpass  Fo=25  Zeta=0.707  Ts=Ts  Initialize=on  Vac_Init=[0 -25 60]  Vdc_Init=Finit  PlotResponse=off  FreqRange=[0, 500, 1]
  Selector : Selector  InputPortWidth=3  IndexOptions=Index vector (dialog)  Indices=2  OutputSizes=1
  Sum : Sum  InputSameDT=on  SaturateOnIntegerOverflow=on  OutDataTypeStr=Inherit: Same as first input
  Unit Delay : UnitDelay  InitialCondition=Finit  SampleTime=Ts  HasFrameUpgradeWarning=on
  abc to dq0 : spsabctodq0Lib/abc to dq0  Alignment=90 degrees behind phase A axis
  Freq : Outport  VectorParamsAs1DForOutWhenUnconnected=off
  wt : Outport  Port=2  VectorParamsAs1DForOutWhenUnconnected=off
  wires:
  Sum/1 -> wt/1
  Selector/1 -> Mean (Variable Frequency)/2  "Vq"
  Second-Order Filter/1 -> Unit Delay/1
  Unit Delay/1 -> Correction for delay/1, Mean (Variable Frequency)/1, Freq/1
  Discrete Rate Limiter/1(Out) -> Second-Order Filter/1
  Gain10/1 -> Discrete Rate Limiter/1(In)
  Discrete PI Controller/1(Out) -> Gain10/1, Discrete-Time Integrator/1  "W"
  Math Function/1 -> abc to dq0/2, Sum/2
  Discrete-Time Integrator/1 -> Math Function/1
  Constant4/1 -> Math Function/2
  abc to dq0/1 -> Selector/1
  Vabc (pu)/1 -> abc to dq0/1
  Mean (Variable Frequency)/1 -> Discrete PI Controller/1(Error)
  Correction for delay/1 -> Sum/1

== system UnifiedPowerFlowController/UPFC Controller/SH Control (STATCOM)/Voltage Regulator ==
  Vref : Inport
  Vmes : Inport  Port=2
  Discrete-Time Integrator : DiscreteIntegrator  InitialCondition=Init  SampleTime=Ts  LimitOutput=on  UpperSaturationLimit=UpperLimit  LowerSaturationLimit=LowerLimit  ICPrevOutput=DiscIntNeverNeededParam  ICPrevScaledInput=DiscIntNeverNeededParam
  Kp4 : Gain  Gain=Kp  SaturateOnIntegerOverflow=on  OutDataTypeStr=Inherit: Same as input  ParamDataTypeStr=Inherit: Same as input
  Kp5 : Gain  Gain=Ki  SaturateOnIntegerOverflow=on  OutDataTypeStr=Inherit: Same as input  ParamDataTypeStr=Inherit: Same as input
  Kp6 : Gain  Gain=Droop  SaturateOnIntegerOverflow=on  OutDataTypeStr=Inherit: Same as input  ParamDataTypeStr=Inherit: Same as input
  Saturation2 : Saturate  UpperLimit=UpperLimit  LowerLimit=LowerLimit
  Sum1 : Sum  Inputs=|-+  InputSameDT=on  SaturateOnIntegerOverflow=on  OutDataTypeStr=Inherit: Same as first input
  Sum6 : Sum  InputSameDT=on  SaturateOnIntegerOverflow=on  OutDataTypeStr=Inherit: Same as first input
  Sum7 : Sum  Inputs=|+-  InputSameDT=on  SaturateOnIntegerOverflow=on  OutDataTypeStr=Inherit: Same as first input
  Unit Delay : UnitDelay  SampleTime=Ts  HasFrameUpgradeWarning=on
  Iqref : Outport  InitialOutput=0  VectorParamsAs1DForOutWhenUnconnected=off
  wires:
  Sum1/1 -> Sum7/1  "Err"
  Vref/1 -> Sum1/2
  Vmes/1 -> Sum1/1
  Unit Delay/1 -> Sum7/2
  Kp6/1 -> Unit Delay/1
  Saturation2/1 -> Kp6/1, Iqref/1  "Iq_Ref"
  Sum7/1 -> Kp4/1, Kp5/1
  Kp5/1 -> Discrete-Time Integrator/1
  Sum6/1 -> Saturation2/1
  Kp4/1 -> Sum6/1
  Discrete-Time Integrator/1 -> Sum6/2

== system UnifiedPowerFlowController/UPFC Controller/SE Control (SSSC)/Firing Pulses Generator/Bridge 1D ==
  wt : Inport  PortDimensions=1
  Alpha : Inport  Port=2  PortDimensions=1
  Sigma : Inport  Port=3  PortDimensions=1
  D_Alpha : Inport  Port=4  PortDimensions=1
  Constant : Constant  Value=-2*pi/3
  Constant1 : Constant  Value=2*pi/3
  Mux1 : Mux  Inputs=[4 4 4]
  Phase A : Subsystem
  Phase B : Subsystem
  Phase C : Subsystem
  Sum : Sum  InputSameDT=on  SaturateOnIntegerOverflow=on  OutDataTypeStr=Inherit: Same as first input
  Sum1 : Sum  InputSameDT=on  SaturateOnIntegerOverflow=on  OutDataTypeStr=Inherit: Same as first input
  Sum2 : Sum  InputSameDT=on  SaturateOnIntegerOverflow=on  OutDataTypeStr=Inherit: Same as first input
  Pulses : Outport  VectorParamsAs1DForOutWhenUnconnected=off
  wires:
  Constant1/1 -> Sum1/2
  Sigma/1 -> Phase A/2(sigma), Phase C/2(sigma), Phase B/2(sigma)
  Alpha/1 -> Sum2/2
  wt/1 -> Sum2/1
  Sum2/1 -> Phase A/1(wt), Sum/1, Sum1/1
  Mux1/1 -> Pulses/1
  Phase A/1(Pulses) -> Mux1/1
  Constant/1 -> Sum/2
  Sum/1 -> Phase B/1(wt)
  Sum1/1 -> Phase C/1(wt)
  D_Alpha/1 -> Phase A/3(D_Alpha), Phase B/3(D_Alpha), Phase C/3(D_Alpha)
  Phase B/1(Pulses) -> Mux1/2
  Phase C/1(Pulses) -> Mux1/3

== system UnifiedPowerFlowController/UPFC Controller/SE Control (SSSC)/Firing Pulses Generator/Bridge 1Y  ==
  wt : Inport  PortDimensions=1
  Alpha : Inport  Port=2  PortDimensions=1
  Sigma : Inport  Port=3  PortDimensions=1
  D_Alpha : Inport  Port=4  PortDimensions=1
  Constant : Constant  Value=-2*pi/3
  Constant1 : Constant  Value=2*pi/3
  Mux1 : Mux  Inputs=[4 4 4]
  Phase A : Subsystem
  Phase B : Subsystem
  Phase C : Subsystem
  Sum : Sum  InputSameDT=on  SaturateOnIntegerOverflow=on  OutDataTypeStr=Inherit: Same as first input
  Sum1 : Sum  InputSameDT=on  SaturateOnIntegerOverflow=on  OutDataTypeStr=Inherit: Same as first input
  Sum2 : Sum  InputSameDT=on  SaturateOnIntegerOverflow=on  OutDataTypeStr=Inherit: Same as first input
  Pulses : Outport  VectorParamsAs1DForOutWhenUnconnected=off
  wires:
  Phase C/1(Pulses) -> Mux1/3
  Phase B/1(Pulses) -> Mux1/2
  D_Alpha/1 -> Phase C/3(D_Alpha), Phase B/3(D_Alpha), Phase A/3(D_Alpha)
  Sum1/1 -> Phase C/1(wt)
  Sum/1 -> Phase B/1(wt)
  Constant/1 -> Sum/2
  Phase A/1(Pulses) -> Mux1/1
  Mux1/1 -> Pulses/1
  Sum2/1 -> Sum1/1, Sum/1, Phase A/1(wt)
  wt/1 -> Sum2/1
  Alpha/1 -> Sum2/2
  Sigma/1 -> Phase B/2(sigma), Phase C/2(sigma), Phase A/2(sigma)
  Constant1/1 -> Sum1/2

== system UnifiedPowerFlowController/UPFC Controller/SE Control (SSSC)/Firing Pulses Generator/Bridge 2D ==
  wt : Inport  PortDimensions=1
  Alpha : Inport  Port=2  PortDimensions=1
  Sigma : Inport  Port=3  PortDimensions=1
  D_Alpha : Inport  Port=4  PortDimensions=1
  Constant : Constant  Value=-2*pi/3
  Constant1 : Constant  Value=2*pi/3
  Mux1 : Mux  Inputs=[4 4 4]
  Phase A : Subsystem
  Phase B : Subsystem
  Phase C : Subsystem
  Sum : Sum  InputSameDT=on  SaturateOnIntegerOverflow=on  OutDataTypeStr=Inherit: Same as first input
  Sum1 : Sum  InputSameDT=on  SaturateOnIntegerOverflow=on  OutDataTypeStr=Inherit: Same as first input
  Sum2 : Sum  InputSameDT=on  SaturateOnIntegerOverflow=on  OutDataTypeStr=Inherit: Same as first input
  Pulses : Outport  VectorParamsAs1DForOutWhenUnconnected=off
  wires:
  Constant1/1 -> Sum1/2
  Sigma/1 -> Phase A/2(sigma), Phase C/2(sigma), Phase B/2(sigma)
  Alpha/1 -> Sum2/2
  wt/1 -> Sum2/1
  Sum2/1 -> Phase A/1(wt), Sum/1, Sum1/1
  Mux1/1 -> Pulses/1
  Phase A/1(Pulses) -> Mux1/1
  Constant/1 -> Sum/2
  Sum/1 -> Phase B/1(wt)
  Sum1/1 -> Phase C/1(wt)
  D_Alpha/1 -> Phase A/3(D_Alpha), Phase B/3(D_Alpha), Phase C/3(D_Alpha)
  Phase B/1(Pulses) -> Mux1/2
  Phase C/1(Pulses) -> Mux1/3

== system UnifiedPowerFlowController/UPFC Controller/SE Control (SSSC)/Firing Pulses Generator/Bridge 2Y ==
  wt : Inport  PortDimensions=1
  Alpha : Inport  Port=2  PortDimensions=1
  Sigma : Inport  Port=3  PortDimensions=1
  D_Alpha : Inport  Port=4  PortDimensions=1
  Constant : Constant  Value=-2*pi/3
  Constant1 : Constant  Value=2*pi/3
  Mux1 : Mux  Inputs=[4 4 4]
  Phase A : Subsystem
  Phase B : Subsystem
  Phase C : Subsystem
  Sum : Sum  InputSameDT=on  SaturateOnIntegerOverflow=on  OutDataTypeStr=Inherit: Same as first input
  Sum1 : Sum  InputSameDT=on  SaturateOnIntegerOverflow=on  OutDataTypeStr=Inherit: Same as first input
  Sum2 : Sum  InputSameDT=on  SaturateOnIntegerOverflow=on  OutDataTypeStr=Inherit: Same as first input
  Pulses : Outport  VectorParamsAs1DForOutWhenUnconnected=off
  wires:
  Phase C/1(Pulses) -> Mux1/3
  Phase B/1(Pulses) -> Mux1/2
  D_Alpha/1 -> Phase C/3(D_Alpha), Phase B/3(D_Alpha), Phase A/3(D_Alpha)
  Sum1/1 -> Phase C/1(wt)
  Sum/1 -> Phase B/1(wt)
  Constant/1 -> Sum/2
  Phase A/1(Pulses) -> Mux1/1
  Mux1/1 -> Pulses/1
  Sum2/1 -> Sum1/1, Sum/1, Phase A/1(wt)
  wt/1 -> Sum2/1
  Alpha/1 -> Sum2/2
  Sigma/1 -> Phase B/2(sigma), Phase C/2(sigma), Phase A/2(sigma)
  Constant1/1 -> Sum1/2

== system UnifiedPowerFlowController/UPFC Controller/SE Control (SSSC)/PLL1/Discrete PI Controller ==
  note: Discrete PID Controller
  note: Pierre Giroux, Gilbert Sybille
      | Power System Simulation Laboratory
      | IREQ, Hydro-Quebc
  Error : Inport  SampleTime=Ts
  Discrete-Time Integrator : DiscreteIntegrator  InitialCondition=Init  SampleTime=Ts  LimitOutput=on  UpperSaturationLimit=UpperLimit  LowerSaturationLimit=LowerLimit  ICPrevOutput=DiscIntNeverNeededParam  ICPrevScaledInput=DiscIntNeverNeededParam
  Kp4 : Gain  Gain=Kp  SaturateOnIntegerOverflow=on  SampleTime=Ts  OutDataTypeStr=Inherit: Same as input  ParamDataTypeStr=Inherit: Same as input
  Kp5 : Gain  Gain=Ki  SaturateOnIntegerOverflow=on  SampleTime=Ts  OutDataTypeStr=Inherit: Same as input  ParamDataTypeStr=Inherit: Same as input
  Saturation2 : Saturate  UpperLimit=UpperLimit  LowerLimit=LowerLimit  SampleTime=Ts
  Sum6 : Sum  InputSameDT=on  SaturateOnIntegerOverflow=on  SampleTime=Ts  OutDataTypeStr=Inherit: Same as first input
  Zero-Order Hold : ZeroOrderHold  SampleTime=Ts
  Out : Outport  SampleTime=Ts  InitialOutput=0  VectorParamsAs1DForOutWhenUnconnected=off
  wires:
  Zero-Order Hold/1 -> Sum6/1
  Saturation2/1 -> Out/1
  Discrete-Time Integrator/1 -> Sum6/2
  Kp4/1 -> Zero-Order Hold/1
  Kp5/1 -> Discrete-Time Integrator/1
  Sum6/1 -> Saturation2/1
  Error/1 -> Kp5/1, Kp4/1

== system UnifiedPowerFlowController/UPFC Controller/SE Control (SSSC)/PLL1/Discrete Rate Limiter ==
  note: Beat Ronner
      | ABB Industrie AG
      | Turgi, Switzerland
  note: Delta(u)
  In : Inport
  Saturation : Saturate  UpperLimit=UpperLimit  LowerLimit=LowerLimit
  Sum : Sum  Inputs=|++  InputSameDT=on  SaturateOnIntegerOverflow=on  OutDataTypeStr=Inherit: Same as first input
  Sum1 : Sum  Inputs=|+-  InputSameDT=on  SaturateOnIntegerOverflow=on  OutDataTypeStr=Inherit: Same as first input
  Unit Delay : UnitDelay  InitialCondition=Vinit  SampleTime=Ts  HasFrameUpgradeWarning=on
  Out : Outport  VectorParamsAs1DForOutWhenUnconnected=off
  wires:
  Unit Delay/1 -> Sum/2, Sum1/2  "y-1"
  Sum/1 -> Unit Delay/1, Out/1  "y"
  Saturation/1 -> Sum/1  "Delta(u)_limit"
  Sum1/1 -> Saturation/1
  In/1 -> Sum1/1  "u"

== system UnifiedPowerFlowController/UPFC Controller/SE Control (UPFC)/Current Regulators/Id PID ==
  note: Pierre Giroux, Gilbert Sybille
      | Power System Simulation Laboratory
      | IREQ, Hydro-Quebc
  note: Discrete PID Controller
  Error : Inport  SampleTime=Ts
  "Derivative " : DiscreteTransferFcn  Numerator=[2 -2]  Denominator=[Ts+2*TcD Ts-2*TcD]  SampleTime=Ts
  Discrete-Time Integrator : DiscreteIntegrator  InitialCondition=Init  SampleTime=Ts  LimitOutput=on  UpperSaturationLimit=UpperLimit  LowerSaturationLimit=LowerLimit  ICPrevOutput=DiscIntNeverNeededParam  ICPrevScaledInput=DiscIntNeverNeededParam
  Kp4 : Gain  Gain=Kp  SaturateOnIntegerOverflow=on  SampleTime=Ts  OutDataTypeStr=Inherit: Same as input  ParamDataTypeStr=Inherit: Same as input
  Kp5 : Gain  Gain=Ki  SaturateOnIntegerOverflow=on  SampleTime=Ts  OutDataTypeStr=Inherit: Same as input  ParamDataTypeStr=Inherit: Same as input
  Kp6 : Gain  Gain=Kd  SaturateOnIntegerOverflow=on  SampleTime=Ts  OutDataTypeStr=Inherit: Same as input  ParamDataTypeStr=Inherit: Same as input
  Saturation2 : Saturate  UpperLimit=UpperLimit  LowerLimit=LowerLimit  SampleTime=Ts
  Sum6 : Sum  Inputs=+++  InputSameDT=on  SaturateOnIntegerOverflow=on  SampleTime=Ts  OutDataTypeStr=Inherit: Same as first input
  Zero-Order Hold : ZeroOrderHold  SampleTime=Ts
  Out : Outport  SampleTime=Ts  InitialOutput=0  VectorParamsAs1DForOutWhenUnconnected=off
  wires:
  Saturation2/1 -> Out/1
  Error/1 -> Kp4/1, Kp5/1, Kp6/1
  Sum6/1 -> Saturation2/1
  Kp5/1 -> Discrete-Time Integrator/1
  Kp6/1 -> "Derivative "/1
  Kp4/1 -> Zero-Order Hold/1
  Discrete-Time Integrator/1 -> Sum6/2
  "Derivative "/1 -> Sum6/3
  Zero-Order Hold/1 -> Sum6/1

== system UnifiedPowerFlowController/UPFC Controller/SE Control (UPFC)/Current Regulators/Id PID1 ==
  note: Pierre Giroux, Gilbert Sybille
      | Power System Simulation Laboratory
      | IREQ, Hydro-Quebc
  note: Discrete PID Controller
  Error : Inport  SampleTime=Ts
  "Derivative " : DiscreteTransferFcn  Numerator=[2 -2]  Denominator=[Ts+2*TcD Ts-2*TcD]  SampleTime=Ts
  Discrete-Time Integrator : DiscreteIntegrator  InitialCondition=Init  SampleTime=Ts  LimitOutput=on  UpperSaturationLimit=UpperLimit  LowerSaturationLimit=LowerLimit  ICPrevOutput=DiscIntNeverNeededParam  ICPrevScaledInput=DiscIntNeverNeededParam
  Kp4 : Gain  Gain=Kp  SaturateOnIntegerOverflow=on  SampleTime=Ts  OutDataTypeStr=Inherit: Same as input  ParamDataTypeStr=Inherit: Same as input
  Kp5 : Gain  Gain=Ki  SaturateOnIntegerOverflow=on  SampleTime=Ts  OutDataTypeStr=Inherit: Same as input  ParamDataTypeStr=Inherit: Same as input
  Kp6 : Gain  Gain=Kd  SaturateOnIntegerOverflow=on  SampleTime=Ts  OutDataTypeStr=Inherit: Same as input  ParamDataTypeStr=Inherit: Same as input
  Saturation2 : Saturate  UpperLimit=UpperLimit  LowerLimit=LowerLimit  SampleTime=Ts
  Sum6 : Sum  Inputs=+++  InputSameDT=on  SaturateOnIntegerOverflow=on  SampleTime=Ts  OutDataTypeStr=Inherit: Same as first input
  Zero-Order Hold : ZeroOrderHold  SampleTime=Ts
  Out : Outport  SampleTime=Ts  InitialOutput=0  VectorParamsAs1DForOutWhenUnconnected=off
  wires:
  Saturation2/1 -> Out/1
  Error/1 -> Kp4/1, Kp5/1, Kp6/1
  Sum6/1 -> Saturation2/1
  Kp5/1 -> Discrete-Time Integrator/1
  Kp6/1 -> "Derivative "/1
  Kp4/1 -> Zero-Order Hold/1
  Discrete-Time Integrator/1 -> Sum6/2
  "Derivative "/1 -> Sum6/3
  Zero-Order Hold/1 -> Sum6/1
